simulink model "Modelo_bergman_mod_U"  (R2024b)
settings: Solver=VariableStepAuto  StartTime=0.0  StopTime=50000  RelTol=1e-3
undefined symbols (not defined in the file): n, p1, p2, p3, Vi
libraries: slpidlib x5
settings Model: Creator=USUARIO  LastModifiedBy=HP
settings SolverCC: AlgebraicLoopSolver=TrustRegion
settings DataIOCC: ReturnWorkspaceOutputs=off
settings DebuggingCC: UnconnectedInputMsg=warning  UnconnectedOutputMsg=warning  UnconnectedLineMsg=warning
settings ModelReferenceCC: EnableRefExpFcnMdlSchedulingChecks=on
settings RTWCC: GPUComputeCapability=3.5

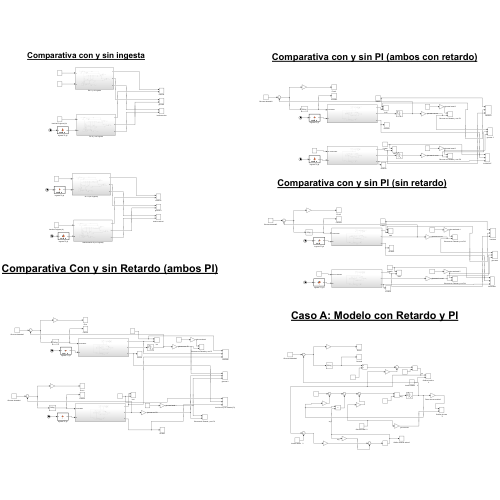
[thumbnail: Simulink's stored preview of the top-level diagram]
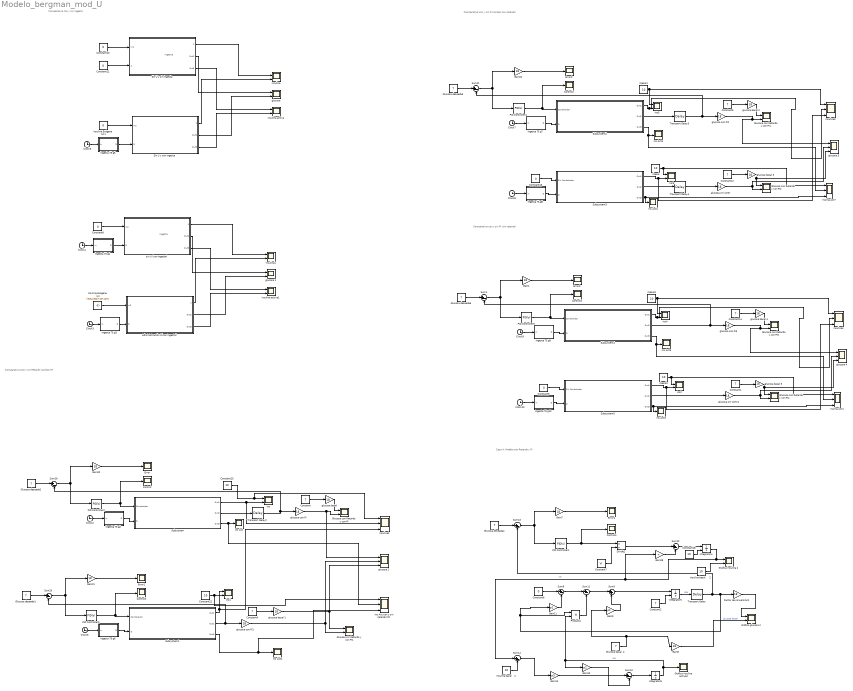
== system Modelo_bergman_mod_U ==
  note: Comparativa con y sin PI (ambos con retardo)
  note: Comparativa con y sin ingesta
  note: ingesta
  note: Comparativa Con y sin Retardo (ambos PI)
  note: Caso A: Modelo con Retardo y PI
  note: ingesta
  note: Comparativa con y sin PI (sin retardo)
  Administración U(con ingesta) : Subsystem
  Clock{2..10} (9 alike) : Clock
  Constant{,1..2,4..5,12,14} (7 alike) : Constant  Value=7
  Constant{3,6,8,10..11,13} (6 alike) : Constant  Value=0
  Constant18 : Constant  Value=10
  Constant22 : Constant  Value=10
  Constant23 : Constant  Value=10
  Constant7 : Constant  Value=Vi
  Control{,1..4} (5 alike) : Scope
  Divide2 : Product  Inputs=*/
  Error{,1..4} (5 alike) : Scope
  Factor de conversión2 : Gain  Gain=18
  Gain{1,7..8,20..22} (6 alike) : Gain  Gain=18
  Gain10 : Gain  Gain=p2
  Gain11 : Gain  Gain=p1
  Gain12 : Gain  Gain=p3
  Gain28 : Gain  Gain=n
  Gain9 : Gain  Gain=p1
  Glucosa basal  2 : Constant  Value=7
  Glucosa con Retardo y con PI{,1..4} (5 alike) : Scope  NumInputPorts=2
  Glucosa deseada{1..5} (5 alike) : Constant  Value=7
  Glucosa sin Retardo y con PI1 : Scope  NumInputPorts=2
  Gráfica glucosa 2 : Scope  NumInputPorts=2
  Gráfica insulina 2 : Scope  NumInputPorts=2
  Gráfica insulina activa2 : Scope
  Ingesta 75 g10 : MATLAB Function  TreatAsAtomicUnit=on
  Ingesta 75 g2 : MATLAB Function  TreatAsAtomicUnit=on
  Ingesta 75 g3 : MATLAB Function  TreatAsAtomicUnit=on
  Ingesta 75 g4 : MATLAB Function  TreatAsAtomicUnit=on
  Ingesta 75 g5 : MATLAB Function  TreatAsAtomicUnit=on
  Ingesta 75 g6 : MATLAB Function  TreatAsAtomicUnit=on
  Ingesta 75 g7 : MATLAB Function  TreatAsAtomicUnit=on
  Ingesta 75 g8 : MATLAB Function  TreatAsAtomicUnit=on
  Ingesta 75 g9 : MATLAB Function  TreatAsAtomicUnit=on
  Ins{,1..5} (6 alike) : Scope  NumInputPorts=2
  Ins Act{,1..5} (6 alike) : Scope
  Ins Act con y sin retardo (PI) : Scope  NumInputPorts=3
  Insulina Exógena (U) : Constant  Value=((5/54)/60)*10*12*5
  Insulina Exógena (U)1 : Constant  Value=0
  Insulina basal      2 : Constant  Value=10
  Insulina basal    2 : Constant  Value=10
  Integrator4 : Integrator  InitialConditionSource=external
  Integrator5 : Integrator  InitialConditionSource=external  InitialCondition=7
  Integrator6 : Integrator
  Inulina Act1 : Scope  NumInputPorts=3
  Inulina Act7 : Scope  NumInputPorts=3
  PID Controller1 : slpidlib/PID Controller  Controller=PID  Form=Parallel  TimeDomain=Continuous-time  UseExternalTs=off  SampleTime=-1  IntegratorMethod=Forward Euler  FilterMethod=Forward Euler  ControllerParametersSource=internal  P=-0.3195  I=-0.3195/2998.95  UseKiTs=off  D=0  UseExternalDerivativeSource=off  N=10  UseFilter=on  TunerSelectOption=Transfer Function Based (PID Tuner App)  InitialConditionSource=internal  InitialConditionForIntegrator=0  InitialConditionForFilter=0  DifferentiatorICPrevScaledInput=0  ExternalReset=none  TrackingMode=off  Kt=1  LimitOutput=off  SatLimitsSource=internal  UpperSaturationLimit=inf  LowerSaturationLimit=-inf  LinearizeAsGain=on  AntiWindupMode=none  Kb=1  LimitIntegrator=off  UpperIntegratorSaturationLimit=inf  LowerIntegratorSaturationLimit=-inf  POutMin=[]  POutMax=[]  IOutMin=[]  IOutMax=[]  DOutMin=[]  DOutMax=[]  NOutMin=[]  NOutMax=[]  SumOutMin=[]  SumOutMax=[]  SaturationOutMin=[]  SaturationOutMax=[]  PParamMin=[]  PParamMax=[]  IParamMin=[]  IParamMax=[]  DParamMin=[]  DParamMax=[]  NParamMin=[]  NParamMax=[]  KbParamMin=[]  KbParamMax=[]  KtParamMin=[]  KtParamMax=[]  KbOutMin=[]  KbOutMax=[]  KtOutMin=[]  KtOutMax=[]  IntegratorOutMin=[]  IntegratorOutMax=[]  FilterOutMin=[]  FilterOutMax=[]  SumI1OutMin=[]  SumI1OutMax=[]  SumI2OutMin=[]  SumI2OutMax=[]  SumI3OutMin=[]  SumI3OutMax=[]  SumI4OutMin=[]  SumI4OutMax=[]  SumDOutMin=[]  SumDOutMax=[]  DifferentiatorOutMin=[]  DifferentiatorOutMax=[]  FilterDiffOutCoefMin=[]  FilterDiffOutCoefMax=[]  ReciprocalOutMin=[]  ReciprocalOutMax=[]  SumDenOutMin=[]  SumDenOutMax=[]  SumNumOutMin=[]  SumNumOutMax=[]  DivideOutMin=[]  DivideOutMax=[]  UdiffTsProdOutMin=[]  UdiffTsProdOutMax=[]  NTsProdOutMin=[]  NTsProdOutMax=[]  UintegralTsProdOutMin=[]  UintegralTsProdOutMax=[]  UngainTsProdOutMin=[]  UngainTsProdOutMax=[]  ClampingZeroOutDataTypeStr=Inherit: Inherit via back propagation  ClampingZeroOutMin=[]  ClampingZeroOutMax=[]  FilterDenConstantOutDataTypeStr=Inherit: Inherit via back propagation  FilterDenConstantOutMin=[]  FilterDenConstantOutMax=[]  PCopyOutDataTypeStr=Inherit: Inherit via back propagation  PCopyOutMin=[]  PCopyOutMax=[]  NCopyOutDataTypeStr=Inherit: Inherit via back propagation  NCopyOutMin=[]  NCopyOutMax=[]  IntegratorContinuousStateAttributes=''  IntegratorStateMustResolveToSignalObject=off  IntegratorRTWStateStorageClass=Auto  FilterContinuousStateAttributes=''  FilterStateMustResolveToSignalObject=off  FilterRTWStateStorageClass=Auto  ParallelPVariant=InternalParameters  IdealPVariant=Disabled  IVariant=InternalParameters  DVariant=InternalParameters  IntegratorVariant=Continuous  SatVariant=Disabled  AWVariant=Passthrough  PCopyVariant=Disabled  TRVariant=Disabled  FdbkBlocksVariant=Forward  IdealPFdbkVariant=Disabled  SatFdbkVariant=Disabled  DerivativeFilterVariant=ContFilter  NVariant=InternalParameters  NCopyVariant=Disabled  FilterICVariant=InternalICsFilter  IntegratorICVariant=InternalICs  ExternalResetVariant=Disabled  TRSumVariant=Passthrough  SumFdbkVariant=Disabled  SumVariant=Sum_PID  TsampFilterVariant=InternalTs  TsampNgainVariant=Passthrough  TsampIntegralVariant=Disabled_SignalSpec  ExternalSaturationOutDataTypeStr=Inherit: Same as second input  DerivativeSourceVariant=ErrorSignal  PreIntVariant=InternalPreInt
  PID Controller2 : slpidlib/PID Controller  Controller=PID  Form=Parallel  TimeDomain=Continuous-time  UseExternalTs=off  SampleTime=-1  IntegratorMethod=Forward Euler  FilterMethod=Forward Euler  ControllerParametersSource=internal  P=-0.3195*0.3  I=-0.3195/2998.95*0.3  UseKiTs=off  D=0  UseExternalDerivativeSource=off  N=10  UseFilter=on  TunerSelectOption=Transfer Function Based (PID Tuner App)  InitialConditionSource=internal  InitialConditionForIntegrator=0  InitialConditionForFilter=0  DifferentiatorICPrevScaledInput=0  ExternalReset=none  TrackingMode=off  Kt=1  LimitOutput=off  SatLimitsSource=internal  UpperSaturationLimit=inf  LowerSaturationLimit=-inf  LinearizeAsGain=on  AntiWindupMode=none  Kb=1  LimitIntegrator=off  UpperIntegratorSaturationLimit=inf  LowerIntegratorSaturationLimit=-inf  POutMin=[]  POutMax=[]  IOutMin=[]  IOutMax=[]  DOutMin=[]  DOutMax=[]  NOutMin=[]  NOutMax=[]  SumOutMin=[]  SumOutMax=[]  SaturationOutMin=[]  SaturationOutMax=[]  PParamMin=[]  PParamMax=[]  IParamMin=[]  IParamMax=[]  DParamMin=[]  DParamMax=[]  NParamMin=[]  NParamMax=[]  KbParamMin=[]  KbParamMax=[]  KtParamMin=[]  KtParamMax=[]  KbOutMin=[]  KbOutMax=[]  KtOutMin=[]  KtOutMax=[]  IntegratorOutMin=[]  IntegratorOutMax=[]  FilterOutMin=[]  FilterOutMax=[]  SumI1OutMin=[]  SumI1OutMax=[]  SumI2OutMin=[]  SumI2OutMax=[]  SumI3OutMin=[]  SumI3OutMax=[]  SumI4OutMin=[]  SumI4OutMax=[]  SumDOutMin=[]  SumDOutMax=[]  DifferentiatorOutMin=[]  DifferentiatorOutMax=[]  FilterDiffOutCoefMin=[]  FilterDiffOutCoefMax=[]  ReciprocalOutMin=[]  ReciprocalOutMax=[]  SumDenOutMin=[]  SumDenOutMax=[]  SumNumOutMin=[]  SumNumOutMax=[]  DivideOutMin=[]  DivideOutMax=[]  UdiffTsProdOutMin=[]  UdiffTsProdOutMax=[]  NTsProdOutMin=[]  NTsProdOutMax=[]  UintegralTsProdOutMin=[]  UintegralTsProdOutMax=[]  UngainTsProdOutMin=[]  UngainTsProdOutMax=[]  ClampingZeroOutDataTypeStr=Inherit: Inherit via back propagation  ClampingZeroOutMin=[]  ClampingZeroOutMax=[]  FilterDenConstantOutDataTypeStr=Inherit: Inherit via back propagation  FilterDenConstantOutMin=[]  FilterDenConstantOutMax=[]  PCopyOutDataTypeStr=Inherit: Inherit via back propagation  PCopyOutMin=[]  PCopyOutMax=[]  NCopyOutDataTypeStr=Inherit: Inherit via back propagation  NCopyOutMin=[]  NCopyOutMax=[]  IntegratorContinuousStateAttributes=''  IntegratorStateMustResolveToSignalObject=off  IntegratorRTWStateStorageClass=Auto  FilterContinuousStateAttributes=''  FilterStateMustResolveToSignalObject=off  FilterRTWStateStorageClass=Auto  ParallelPVariant=InternalParameters  IdealPVariant=Disabled  IVariant=InternalParameters  DVariant=InternalParameters  IntegratorVariant=Continuous  SatVariant=Disabled  AWVariant=Passthrough  PCopyVariant=Disabled  TRVariant=Disabled  FdbkBlocksVariant=Forward  IdealPFdbkVariant=Disabled  SatFdbkVariant=Disabled  DerivativeFilterVariant=ContFilter  NVariant=InternalParameters  NCopyVariant=Disabled  FilterICVariant=InternalICsFilter  IntegratorICVariant=InternalICs  ExternalResetVariant=Disabled  TRSumVariant=Passthrough  SumFdbkVariant=Disabled  SumVariant=Sum_PID  TsampFilterVariant=InternalTs  TsampNgainVariant=Passthrough  TsampIntegralVariant=Disabled_SignalSpec  ExternalSaturationOutDataTypeStr=Inherit: Same as second input  DerivativeSourceVariant=ErrorSignal  PreIntVariant=InternalPreInt
  PID Controller3 : slpidlib/PID Controller  Controller=PID  Form=Parallel  TimeDomain=Continuous-time  UseExternalTs=off  SampleTime=-1  IntegratorMethod=Forward Euler  FilterMethod=Forward Euler  ControllerParametersSource=internal  P=-0.3195*0.3  I=-0.3195/2998.95*0.3  UseKiTs=off  D=0  UseExternalDerivativeSource=off  N=10  UseFilter=on  TunerSelectOption=Transfer Function Based (PID Tuner App)  InitialConditionSource=internal  InitialConditionForIntegrator=0  InitialConditionForFilter=0  DifferentiatorICPrevScaledInput=0  ExternalReset=none  TrackingMode=off  Kt=1  LimitOutput=off  SatLimitsSource=internal  UpperSaturationLimit=inf  LowerSaturationLimit=-inf  LinearizeAsGain=on  AntiWindupMode=none  Kb=1  LimitIntegrator=off  UpperIntegratorSaturationLimit=inf  LowerIntegratorSaturationLimit=-inf  POutMin=[]  POutMax=[]  IOutMin=[]  IOutMax=[]  DOutMin=[]  DOutMax=[]  NOutMin=[]  NOutMax=[]  SumOutMin=[]  SumOutMax=[]  SaturationOutMin=[]  SaturationOutMax=[]  PParamMin=[]  PParamMax=[]  IParamMin=[]  IParamMax=[]  DParamMin=[]  DParamMax=[]  NParamMin=[]  NParamMax=[]  KbParamMin=[]  KbParamMax=[]  KtParamMin=[]  KtParamMax=[]  KbOutMin=[]  KbOutMax=[]  KtOutMin=[]  KtOutMax=[]  IntegratorOutMin=[]  IntegratorOutMax=[]  FilterOutMin=[]  FilterOutMax=[]  SumI1OutMin=[]  SumI1OutMax=[]  SumI2OutMin=[]  SumI2OutMax=[]  SumI3OutMin=[]  SumI3OutMax=[]  SumI4OutMin=[]  SumI4OutMax=[]  SumDOutMin=[]  SumDOutMax=[]  DifferentiatorOutMin=[]  DifferentiatorOutMax=[]  FilterDiffOutCoefMin=[]  FilterDiffOutCoefMax=[]  ReciprocalOutMin=[]  ReciprocalOutMax=[]  SumDenOutMin=[]  SumDenOutMax=[]  SumNumOutMin=[]  SumNumOutMax=[]  DivideOutMin=[]  DivideOutMax=[]  UdiffTsProdOutMin=[]  UdiffTsProdOutMax=[]  NTsProdOutMin=[]  NTsProdOutMax=[]  UintegralTsProdOutMin=[]  UintegralTsProdOutMax=[]  UngainTsProdOutMin=[]  UngainTsProdOutMax=[]  ClampingZeroOutDataTypeStr=Inherit: Inherit via back propagation  ClampingZeroOutMin=[]  ClampingZeroOutMax=[]  FilterDenConstantOutDataTypeStr=Inherit: Inherit via back propagation  FilterDenConstantOutMin=[]  FilterDenConstantOutMax=[]  PCopyOutDataTypeStr=Inherit: Inherit via back propagation  PCopyOutMin=[]  PCopyOutMax=[]  NCopyOutDataTypeStr=Inherit: Inherit via back propagation  NCopyOutMin=[]  NCopyOutMax=[]  IntegratorContinuousStateAttributes=''  IntegratorStateMustResolveToSignalObject=off  IntegratorRTWStateStorageClass=Auto  FilterContinuousStateAttributes=''  FilterStateMustResolveToSignalObject=off  FilterRTWStateStorageClass=Auto  ParallelPVariant=InternalParameters  IdealPVariant=Disabled  IVariant=InternalParameters  DVariant=InternalParameters  IntegratorVariant=Continuous  SatVariant=Disabled  AWVariant=Passthrough  PCopyVariant=Disabled  TRVariant=Disabled  FdbkBlocksVariant=Forward  IdealPFdbkVariant=Disabled  SatFdbkVariant=Disabled  DerivativeFilterVariant=ContFilter  NVariant=InternalParameters  NCopyVariant=Disabled  FilterICVariant=InternalICsFilter  IntegratorICVariant=InternalICs  ExternalResetVariant=Disabled  TRSumVariant=Passthrough  SumFdbkVariant=Disabled  SumVariant=Sum_PID  TsampFilterVariant=InternalTs  TsampNgainVariant=Passthrough  TsampIntegralVariant=Disabled_SignalSpec  ExternalSaturationOutDataTypeStr=Inherit: Same as second input  DerivativeSourceVariant=ErrorSignal  PreIntVariant=InternalPreInt
  PID Controller4 : slpidlib/PID Controller  Controller=PID  Form=Parallel  TimeDomain=Continuous-time  UseExternalTs=off  SampleTime=-1  IntegratorMethod=Forward Euler  FilterMethod=Forward Euler  ControllerParametersSource=internal  P=-0.3195  I=-0.3195/2998.95  UseKiTs=off  D=0  UseExternalDerivativeSource=off  N=10  UseFilter=on  TunerSelectOption=Transfer Function Based (PID Tuner App)  InitialConditionSource=internal  InitialConditionForIntegrator=0  InitialConditionForFilter=0  DifferentiatorICPrevScaledInput=0  ExternalReset=none  TrackingMode=off  Kt=1  LimitOutput=off  SatLimitsSource=internal  UpperSaturationLimit=inf  LowerSaturationLimit=-inf  LinearizeAsGain=on  AntiWindupMode=none  Kb=1  LimitIntegrator=off  UpperIntegratorSaturationLimit=inf  LowerIntegratorSaturationLimit=-inf  POutMin=[]  POutMax=[]  IOutMin=[]  IOutMax=[]  DOutMin=[]  DOutMax=[]  NOutMin=[]  NOutMax=[]  SumOutMin=[]  SumOutMax=[]  SaturationOutMin=[]  SaturationOutMax=[]  PParamMin=[]  PParamMax=[]  IParamMin=[]  IParamMax=[]  DParamMin=[]  DParamMax=[]  NParamMin=[]  NParamMax=[]  KbParamMin=[]  KbParamMax=[]  KtParamMin=[]  KtParamMax=[]  KbOutMin=[]  KbOutMax=[]  KtOutMin=[]  KtOutMax=[]  IntegratorOutMin=[]  IntegratorOutMax=[]  FilterOutMin=[]  FilterOutMax=[]  SumI1OutMin=[]  SumI1OutMax=[]  SumI2OutMin=[]  SumI2OutMax=[]  SumI3OutMin=[]  SumI3OutMax=[]  SumI4OutMin=[]  SumI4OutMax=[]  SumDOutMin=[]  SumDOutMax=[]  DifferentiatorOutMin=[]  DifferentiatorOutMax=[]  FilterDiffOutCoefMin=[]  FilterDiffOutCoefMax=[]  ReciprocalOutMin=[]  ReciprocalOutMax=[]  SumDenOutMin=[]  SumDenOutMax=[]  SumNumOutMin=[]  SumNumOutMax=[]  DivideOutMin=[]  DivideOutMax=[]  UdiffTsProdOutMin=[]  UdiffTsProdOutMax=[]  NTsProdOutMin=[]  NTsProdOutMax=[]  UintegralTsProdOutMin=[]  UintegralTsProdOutMax=[]  UngainTsProdOutMin=[]  UngainTsProdOutMax=[]  ClampingZeroOutDataTypeStr=Inherit: Inherit via back propagation  ClampingZeroOutMin=[]  ClampingZeroOutMax=[]  FilterDenConstantOutDataTypeStr=Inherit: Inherit via back propagation  FilterDenConstantOutMin=[]  FilterDenConstantOutMax=[]  PCopyOutDataTypeStr=Inherit: Inherit via back propagation  PCopyOutMin=[]  PCopyOutMax=[]  NCopyOutDataTypeStr=Inherit: Inherit via back propagation  NCopyOutMin=[]  NCopyOutMax=[]  IntegratorContinuousStateAttributes=''  IntegratorStateMustResolveToSignalObject=off  IntegratorRTWStateStorageClass=Auto  FilterContinuousStateAttributes=''  FilterStateMustResolveToSignalObject=off  FilterRTWStateStorageClass=Auto  ParallelPVariant=InternalParameters  IdealPVariant=Disabled  IVariant=InternalParameters  DVariant=InternalParameters  IntegratorVariant=Continuous  SatVariant=Disabled  AWVariant=Passthrough  PCopyVariant=Disabled  TRVariant=Disabled  FdbkBlocksVariant=Forward  IdealPFdbkVariant=Disabled  SatFdbkVariant=Disabled  DerivativeFilterVariant=ContFilter  NVariant=InternalParameters  NCopyVariant=Disabled  FilterICVariant=InternalICsFilter  IntegratorICVariant=InternalICs  ExternalResetVariant=Disabled  TRSumVariant=Passthrough  SumFdbkVariant=Disabled  SumVariant=Sum_PID  TsampFilterVariant=InternalTs  TsampNgainVariant=Passthrough  TsampIntegralVariant=Disabled_SignalSpec  ExternalSaturationOutDataTypeStr=Inherit: Same as second input  DerivativeSourceVariant=ErrorSignal  PreIntVariant=InternalPreInt
  PID Controller5 : slpidlib/PID Controller  Controller=PID  Form=Parallel  TimeDomain=Continuous-time  UseExternalTs=off  SampleTime=-1  IntegratorMethod=Forward Euler  FilterMethod=Forward Euler  ControllerParametersSource=internal  P=-0.3195  I=-0.3195/2998.95  UseKiTs=off  D=0  UseExternalDerivativeSource=off  N=10  UseFilter=on  TunerSelectOption=Transfer Function Based (PID Tuner App)  InitialConditionSource=internal  InitialConditionForIntegrator=0  InitialConditionForFilter=0  DifferentiatorICPrevScaledInput=0  ExternalReset=none  TrackingMode=off  Kt=1  LimitOutput=off  SatLimitsSource=internal  UpperSaturationLimit=inf  LowerSaturationLimit=-inf  LinearizeAsGain=on  AntiWindupMode=none  Kb=1  LimitIntegrator=off  UpperIntegratorSaturationLimit=inf  LowerIntegratorSaturationLimit=-inf  POutMin=[]  POutMax=[]  IOutMin=[]  IOutMax=[]  DOutMin=[]  DOutMax=[]  NOutMin=[]  NOutMax=[]  SumOutMin=[]  SumOutMax=[]  SaturationOutMin=[]  SaturationOutMax=[]  PParamMin=[]  PParamMax=[]  IParamMin=[]  IParamMax=[]  DParamMin=[]  DParamMax=[]  NParamMin=[]  NParamMax=[]  KbParamMin=[]  KbParamMax=[]  KtParamMin=[]  KtParamMax=[]  KbOutMin=[]  KbOutMax=[]  KtOutMin=[]  KtOutMax=[]  IntegratorOutMin=[]  IntegratorOutMax=[]  FilterOutMin=[]  FilterOutMax=[]  SumI1OutMin=[]  SumI1OutMax=[]  SumI2OutMin=[]  SumI2OutMax=[]  SumI3OutMin=[]  SumI3OutMax=[]  SumI4OutMin=[]  SumI4OutMax=[]  SumDOutMin=[]  SumDOutMax=[]  DifferentiatorOutMin=[]  DifferentiatorOutMax=[]  FilterDiffOutCoefMin=[]  FilterDiffOutCoefMax=[]  ReciprocalOutMin=[]  ReciprocalOutMax=[]  SumDenOutMin=[]  SumDenOutMax=[]  SumNumOutMin=[]  SumNumOutMax=[]  DivideOutMin=[]  DivideOutMax=[]  UdiffTsProdOutMin=[]  UdiffTsProdOutMax=[]  NTsProdOutMin=[]  NTsProdOutMax=[]  UintegralTsProdOutMin=[]  UintegralTsProdOutMax=[]  UngainTsProdOutMin=[]  UngainTsProdOutMax=[]  ClampingZeroOutDataTypeStr=Inherit: Inherit via back propagation  ClampingZeroOutMin=[]  ClampingZeroOutMax=[]  FilterDenConstantOutDataTypeStr=Inherit: Inherit via back propagation  FilterDenConstantOutMin=[]  FilterDenConstantOutMax=[]  PCopyOutDataTypeStr=Inherit: Inherit via back propagation  PCopyOutMin=[]  PCopyOutMax=[]  NCopyOutDataTypeStr=Inherit: Inherit via back propagation  NCopyOutMin=[]  NCopyOutMax=[]  IntegratorContinuousStateAttributes=''  IntegratorStateMustResolveToSignalObject=off  IntegratorRTWStateStorageClass=Auto  FilterContinuousStateAttributes=''  FilterStateMustResolveToSignalObject=off  FilterRTWStateStorageClass=Auto  ParallelPVariant=InternalParameters  IdealPVariant=Disabled  IVariant=InternalParameters  DVariant=InternalParameters  IntegratorVariant=Continuous  SatVariant=Disabled  AWVariant=Passthrough  PCopyVariant=Disabled  TRVariant=Disabled  FdbkBlocksVariant=Forward  IdealPFdbkVariant=Disabled  SatFdbkVariant=Disabled  DerivativeFilterVariant=ContFilter  NVariant=InternalParameters  NCopyVariant=Disabled  FilterICVariant=InternalICsFilter  IntegratorICVariant=InternalICs  ExternalResetVariant=Disabled  TRSumVariant=Passthrough  SumFdbkVariant=Disabled  SumVariant=Sum_PID  TsampFilterVariant=InternalTs  TsampNgainVariant=Passthrough  TsampIntegralVariant=Disabled_SignalSpec  ExternalSaturationOutDataTypeStr=Inherit: Same as second input  DerivativeSourceVariant=ErrorSignal  PreIntVariant=InternalPreInt
  Product2 : Product
  Sin U y con Ingesta : Subsystem
  Sin U y sin ingesta : Subsystem
  Subsystem : Subsystem
  Subsystem1 : Subsystem
  Subsystem2 : Subsystem
  Subsystem3 : Subsystem
  Subsystem4 : Subsystem
  Subsystem5 : Subsystem
  Sum{1,8,10..14,20..21,29} (10 alike) : Sum  Inputs=|+-
  Sum9 : Sum  Inputs=|++
  Transport Delay : TransportDelay  DelayTime=900
  Transport Delay2 : TransportDelay  DelayTime=900  InitialOutput=7
  Transport Delay3 : TransportDelay  DelayTime=600  InitialOutput=7
  Transport Delay4 : TransportDelay  DelayTime=600  InitialOutput=7
  "glucosa " : Scope  NumInputPorts=2
  glucosa 1 : Scope  NumInputPorts=2
  glucosa 2 : Scope  NumInputPorts=3
  glucosa 3 : Scope  NumInputPorts=3
  glucosa 4 : Scope  NumInputPorts=3
  glucosa basal {,1..5} (6 alike) : Gain  Gain=18
  glucosa con PI{,1..3} (4 alike) : Gain  Gain=18
  glucosa sin contr : Gain  Gain=18
  glucosa sin contr1 : Gain  Gain=18
  i basal{,1..3} (4 alike) : Constant  Value=10
  insulina : Scope  NumInputPorts=2
  insulina activa : Scope  NumInputPorts=2
  insulina activa1 : Scope  NumInputPorts=2
  insulina1 : Scope  NumInputPorts=2
  insulina2 : Scope  NumInputPorts=3
  insulina3 : Scope  NumInputPorts=3
  insulina4 : Scope  NumInputPorts=3
  sin U (con Ingesta) : Subsystem
  wires:
  Constant6/1 -> Sum8/1
  Divide2/1 -> Sum12/1
  Gain11/1 -> Sum8/2
  Product2/1 -> Sum11/2
  Factor de conversión2/1 -> Gráfica glucosa 2/1
  Glucosa basal  2/1 -> Gain9/1, Gain8/1
  Sum10/1 -> Integrator6/1
  Constant18/1 -> Integrator4/2
  Glucosa deseada4/1 -> Sum13/1
  PID Controller1/1 -> Control4/1, Divide2/1
  Sum8/1 -> Sum11/1
  Gain8/1 -> Gráfica glucosa 2/2  "glucosa basal"
  Sum11/1 -> Sum9/1
  Sum13/1 -> PID Controller1/1, Gain7/1
  Insulina basal    2/1 -> Sum14/2
  Sum9/1 -> Integrator5/1
  Integrator4/1 -> Gráfica insulina 2/1, Sum14/1, Gain28/1  "I(t)"
  Integrator5/1 -> Transport Delay/1  "G(t)"
  Insulina basal      2/1 -> Gráfica insulina 2/2
  Gain10/1 -> Sum10/2
  Sum14/1 -> Gain12/1
  Sum12/1 -> Integrator4/1
  Gain7/1 -> Error4/1
  Gain12/1 -> Sum10/1
  Integrator6/1 -> Product2/2, Gain10/1, Gráfica insulina activa2/1  "X(t)"
  Constant7/1 -> Divide2/2
  Constant2/1 -> Integrator5/2
  Gain28/1 -> Sum12/2
  Gain9/1 -> Sum9/2
  Constant8/1 -> sin U (con Ingesta)/1(In2)
  Insulina Exógena (U)/1 -> Administración U(con ingesta)/1(In2)
  sin U (con Ingesta)/2(Out2) -> glucosa 1/1
  Administración U(con ingesta)/2(Out2) -> glucosa 1/2
  Administración U(con ingesta)/1(1) -> insulina1/2
  sin U (con Ingesta)/1(1) -> insulina1/1
  Clock4/1 -> Ingesta 75 g4/1(in)
  Ingesta 75 g3/1(D) -> Administración U(con ingesta)/2(D)
  Clock3/1 -> Ingesta 75 g3/1(in)
  Ingesta 75 g4/1(D) -> sin U (con Ingesta)/2(D)
  Administración U(con ingesta)/3(Out3) -> insulina activa1/2
  sin U (con Ingesta)/3(Out3) -> insulina activa1/1
  Sin U y sin ingesta/3(Out3) -> insulina activa/1
  Sin U y con Ingesta/1(1) -> insulina/2
  Ingesta 75 g5/1(D) -> Sin U y con Ingesta/2(D)
  Sin U y con Ingesta/3(Out3) -> insulina activa/2
  Constant10/1 -> Sin U y sin ingesta/1(In2)
  Insulina Exógena (U)1/1 -> Sin U y con Ingesta/1(In2)
  Clock5/1 -> Ingesta 75 g5/1(in)
  Sin U y sin ingesta/1(1) -> insulina/1
  Sin U y con Ingesta/2(Out2) -> "glucosa "/2
  Sin U y sin ingesta/2(Out2) -> "glucosa "/1
  Constant11/1 -> Sin U y sin ingesta/2(2)
  Clock2/1 -> Ingesta 75 g2/1(in)
  Ingesta 75 g2/1(D) -> Subsystem/2(D)
  PID Controller2/1 -> Control/1, Subsystem/1(Controlador)
  Glucosa deseada2/1 -> Sum29/1
  Gain20/1 -> Error/1
  Sum29/1 -> PID Controller2/1, Gain20/1
  Transport Delay2/1 -> Sum29/2, glucosa con PI/1
  glucosa con PI/1 -> glucosa 2/1, Glucosa con Retardo y con PI/2
  Subsystem/2(Out2) -> Transport Delay2/1
  Constant/1 -> "glucosa basal "/1
  "glucosa basal "/1 -> Glucosa con Retardo y con PI/1
  PID Controller3/1 -> Control1/1, Subsystem1/1(Controlador)
  Gain21/1 -> Error1/1
  Constant4/1 -> glucosa basal 1/1
  glucosa con PI1/1 -> glucosa 2/2, Glucosa sin Retardo y con PI1/2
  Sum20/1 -> PID Controller3/1, Gain21/1
  Glucosa deseada1/1 -> Sum20/1
  glucosa basal 1/1 -> glucosa 2/3, Glucosa sin Retardo y con PI1/1
  Clock6/1 -> Ingesta 75 g6/1(in)
  Ingesta 75 g6/1(D) -> Subsystem1/2(D)
  Subsystem1/2(Out2) -> Sum20/2, glucosa con PI1/1
  PID Controller4/1 -> Control2/1, Subsystem2/1(Controlador)
  Gain22/1 -> Error2/1
  Constant5/1 -> glucosa basal 2/1
  glucosa con PI2/1 -> glucosa 3/1, Glucosa con Retardo y con PI1/2
  Sum21/1 -> PID Controller4/1, Gain22/1
  Transport Delay3/1 -> Sum21/2, glucosa con PI2/1
  Subsystem2/2(Out2) -> Transport Delay3/1
  Glucosa deseada3/1 -> Sum21/1
  glucosa basal 2/1 -> Glucosa con Retardo y con PI1/1
  Clock7/1 -> Ingesta 75 g7/1(in)
  Ingesta 75 g7/1(D) -> Subsystem2/2(D)
  Constant12/1 -> glucosa basal 3/1
  glucosa sin contr/1 -> glucosa 3/2, Glucosa con Retardo y con PI2/2
  Transport Delay4/1 -> glucosa sin contr/1
  Subsystem3/2(Out2) -> Transport Delay4/1
  glucosa basal 3/1 -> glucosa 3/3, Glucosa con Retardo y con PI2/1
  Clock8/1 -> Ingesta 75 g8/1(in)
  Ingesta 75 g8/1(D) -> Subsystem3/2(D)
  Constant13/1 -> Subsystem3/1(Sin Controlador)
  Subsystem/3(Out3) -> Ins Act con y sin retardo (PI)/2, Ins Act/1
  Subsystem/1(Out1) -> insulina2/2, Ins/2
  Subsystem1/1(Out1) -> insulina2/3, Ins1/1
  Subsystem1/3(Out3) -> Ins Act1/1, Ins Act con y sin retardo (PI)/3
  Constant22/1 -> Ins Act con y sin retardo (PI)/1, Ins1/2
  Constant23/1 -> insulina2/1, Ins/1
  Subsystem2/1(Out1) -> insulina3/2, Ins5/2
  Subsystem2/3(Out3) -> Inulina Act7/2, Ins Act4/1
  Subsystem3/1(Out1) -> insulina3/3, Ins3/2
  Subsystem3/3(Out3) -> Inulina Act7/3, Ins Act2/1
  i basal/1 -> Ins3/1, Inulina Act7/1
  i basal1/1 -> insulina3/1, Ins5/1
  Subsystem4/1(Out1) -> insulina4/2, Ins4/2
  glucosa con PI3/1 -> glucosa 4/1, Glucosa con Retardo y con PI3/2
  glucosa basal 5/1 -> glucosa 4/3, Glucosa con Retardo y con PI4/1
  i basal3/1 -> insulina4/1, Ins4/1
  Subsystem5/2(Out2) -> glucosa sin contr1/1
  Glucosa deseada5/1 -> Sum1/1
  Subsystem4/3(Out3) -> Inulina Act1/2, Ins Act5/1
  Subsystem4/2(Out2) -> Sum1/2, glucosa con PI3/1
  Subsystem5/1(Out1) -> insulina4/3, Ins2/2
  Gain1/1 -> Error3/1
  Sum1/1 -> PID Controller5/1, Gain1/1
  Constant1/1 -> glucosa basal 5/1
  i basal2/1 -> Ins2/1, Inulina Act1/1
  glucosa sin contr1/1 -> glucosa 4/2, Glucosa con Retardo y con PI4/2
  Clock9/1 -> Ingesta 75 g9/1(in)
  PID Controller5/1 -> Control3/1, Subsystem4/1(Controlador)
  Ingesta 75 g9/1(D) -> Subsystem4/2(D)
  Clock10/1 -> Ingesta 75 g10/1(in)
  Subsystem5/3(Out3) -> Inulina Act1/3, Ins Act3/1
  Constant14/1 -> glucosa basal 4/1
  Constant3/1 -> Subsystem5/1(Sin Controlador)
  Ingesta 75 g10/1(D) -> Subsystem5/2(D)
  glucosa basal 4/1 -> Glucosa con Retardo y con PI3/1
  Transport Delay/1 -> Sum13/2, Factor de conversión2/1, Gain11/1, Product2/1

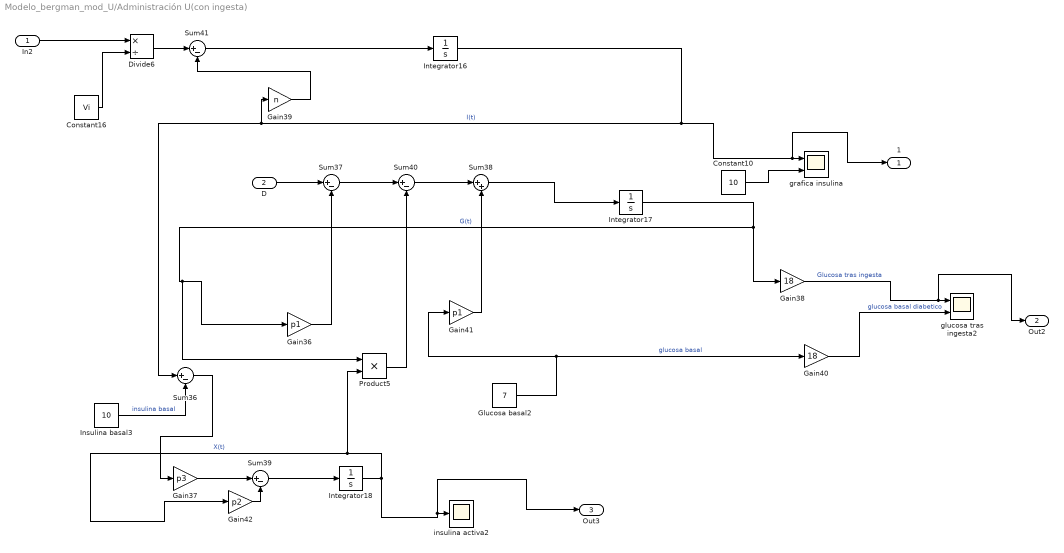
== system Modelo_bergman_mod_U/Administración U(con ingesta) ==
  In2 : Inport
  D : Inport  Port=2
  Constant10 : Constant  Value=10
  Constant16 : Constant  Value=Vi
  Divide6 : Product  Inputs=*/
  Gain36 : Gain  Gain=p1
  Gain37 : Gain  Gain=p3
  Gain38 : Gain  Gain=18
  Gain39 : Gain  Gain=n
  Gain40 : Gain  Gain=18
  Gain41 : Gain  Gain=p1
  Gain42 : Gain  Gain=p2
  Glucosa basal2 : Constant  Value=7
  Insulina basal3 : Constant  Value=10
  Integrator16 : Integrator  InitialCondition=10
  Integrator17 : Integrator  InitialCondition=7
  Integrator18 : Integrator
  Product5 : Product
  Sum{36..37,39..41} (5 alike) : Sum  Inputs=|+-
  Sum38 : Sum  Inputs=|++
  glucosa tras ingesta2 : Scope  NumInputPorts=2
  grafica insulina : Scope  NumInputPorts=2
  insulina activa2 : Scope
  1 : Outport
  Out2 : Outport  Port=2
  Out3 : Outport  Port=3
  wires:
  Integrator18/1 -> Out3/1, insulina activa2/1, Product5/2, Gain42/1  "X(t)"
  Integrator17/1 -> Gain38/1, Product5/1, Gain36/1  "G(t)"
  Gain39/1 -> Sum41/2
  Glucosa basal2/1 -> Gain41/1, Gain40/1  "glucosa basal"
  Integrator16/1 -> Sum36/1, Gain39/1, 1/1, grafica insulina/1  "I(t)"
  Constant10/1 -> grafica insulina/2
  Gain42/1 -> Sum39/2
  D/1 -> Sum37/1
  Sum37/1 -> Sum40/1
  Sum39/1 -> Integrator18/1
  Gain40/1 -> glucosa tras ingesta2/2  "glucosa basal diabetico"
  Sum40/1 -> Sum38/1
  In2/1 -> Divide6/1
  Gain36/1 -> Sum37/2
  Gain38/1 -> Out2/1, glucosa tras ingesta2/1  "Glucosa tras ingesta"
  Sum36/1 -> Gain37/1
  Gain41/1 -> Sum38/2
  Gain37/1 -> Sum39/1
  Sum41/1 -> Integrator16/1
  Sum38/1 -> Integrator17/1
  Insulina basal3/1 -> Sum36/2  "insulina basal"
  Divide6/1 -> Sum41/1
  Constant16/1 -> Divide6/2
  Product5/1 -> Sum40/2

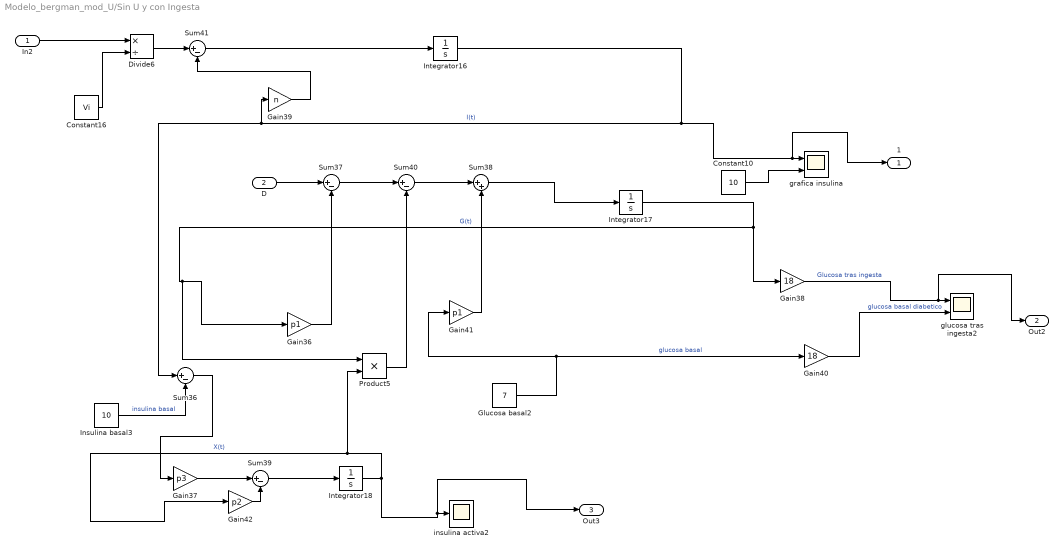
== system Modelo_bergman_mod_U/Sin U y con Ingesta ==
  In2 : Inport
  D : Inport  Port=2
  Constant10 : Constant  Value=10
  Constant16 : Constant  Value=Vi
  Divide6 : Product  Inputs=*/
  Gain36 : Gain  Gain=p1
  Gain37 : Gain  Gain=p3
  Gain38 : Gain  Gain=18
  Gain39 : Gain  Gain=n
  Gain40 : Gain  Gain=18
  Gain41 : Gain  Gain=p1
  Gain42 : Gain  Gain=p2
  Glucosa basal2 : Constant  Value=7
  Insulina basal3 : Constant  Value=10
  Integrator16 : Integrator  InitialCondition=10
  Integrator17 : Integrator  InitialCondition=7
  Integrator18 : Integrator
  Product5 : Product
  Sum{36..37,39..41} (5 alike) : Sum  Inputs=|+-
  Sum38 : Sum  Inputs=|++
  glucosa tras ingesta2 : Scope  NumInputPorts=2
  grafica insulina : Scope  NumInputPorts=2
  insulina activa2 : Scope
  1 : Outport
  Out2 : Outport  Port=2
  Out3 : Outport  Port=3
  wires:
  Integrator18/1 -> Out3/1, insulina activa2/1, Product5/2, Gain42/1  "X(t)"
  Integrator17/1 -> Gain38/1, Product5/1, Gain36/1  "G(t)"
  Gain39/1 -> Sum41/2
  Glucosa basal2/1 -> Gain41/1, Gain40/1  "glucosa basal"
  Integrator16/1 -> Sum36/1, Gain39/1, 1/1, grafica insulina/1  "I(t)"
  Constant10/1 -> grafica insulina/2
  Gain42/1 -> Sum39/2
  D/1 -> Sum37/1
  Sum37/1 -> Sum40/1
  Sum39/1 -> Integrator18/1
  Gain40/1 -> glucosa tras ingesta2/2  "glucosa basal diabetico"
  Sum40/1 -> Sum38/1
  In2/1 -> Divide6/1
  Gain36/1 -> Sum37/2
  Gain38/1 -> Out2/1, glucosa tras ingesta2/1  "Glucosa tras ingesta"
  Sum36/1 -> Gain37/1
  Gain41/1 -> Sum38/2
  Gain37/1 -> Sum39/1
  Sum41/1 -> Integrator16/1
  Sum38/1 -> Integrator17/1
  Insulina basal3/1 -> Sum36/2  "insulina basal"
  Divide6/1 -> Sum41/1
  Constant16/1 -> Divide6/2
  Product5/1 -> Sum40/2

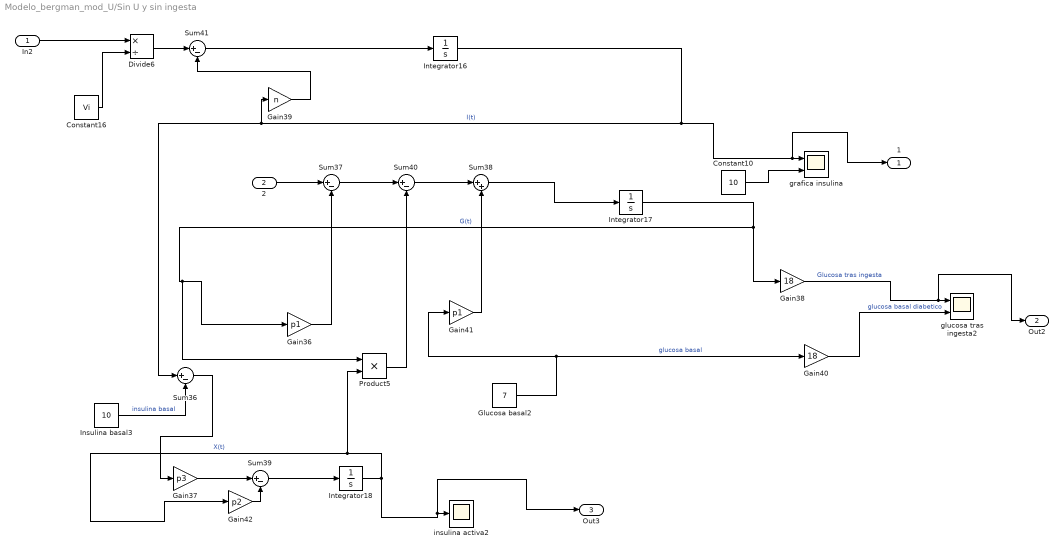
== system Modelo_bergman_mod_U/Sin U y sin ingesta ==
  In2 : Inport
  2 : Inport  Port=2
  Constant10 : Constant  Value=10
  Constant16 : Constant  Value=Vi
  Divide6 : Product  Inputs=*/
  Gain36 : Gain  Gain=p1
  Gain37 : Gain  Gain=p3
  Gain38 : Gain  Gain=18
  Gain39 : Gain  Gain=n
  Gain40 : Gain  Gain=18
  Gain41 : Gain  Gain=p1
  Gain42 : Gain  Gain=p2
  Glucosa basal2 : Constant  Value=7
  Insulina basal3 : Constant  Value=10
  Integrator16 : Integrator  InitialCondition=10
  Integrator17 : Integrator  InitialCondition=7
  Integrator18 : Integrator
  Product5 : Product
  Sum{36..37,39..41} (5 alike) : Sum  Inputs=|+-
  Sum38 : Sum  Inputs=|++
  glucosa tras ingesta2 : Scope  NumInputPorts=2
  grafica insulina : Scope  NumInputPorts=2
  insulina activa2 : Scope
  1 : Outport
  Out2 : Outport  Port=2
  Out3 : Outport  Port=3
  wires:
  Integrator18/1 -> Out3/1, insulina activa2/1, Product5/2, Gain42/1  "X(t)"
  Integrator17/1 -> Gain38/1, Product5/1, Gain36/1  "G(t)"
  Gain39/1 -> Sum41/2
  Glucosa basal2/1 -> Gain41/1, Gain40/1  "glucosa basal"
  Integrator16/1 -> Sum36/1, Gain39/1, 1/1, grafica insulina/1  "I(t)"
  Constant10/1 -> grafica insulina/2
  Gain42/1 -> Sum39/2
  2/1 -> Sum37/1
  Sum37/1 -> Sum40/1
  Sum39/1 -> Integrator18/1
  Gain40/1 -> glucosa tras ingesta2/2  "glucosa basal diabetico"
  Sum40/1 -> Sum38/1
  In2/1 -> Divide6/1
  Gain36/1 -> Sum37/2
  Gain38/1 -> Out2/1, glucosa tras ingesta2/1  "Glucosa tras ingesta"
  Sum36/1 -> Gain37/1
  Gain41/1 -> Sum38/2
  Gain37/1 -> Sum39/1
  Sum41/1 -> Integrator16/1
  Sum38/1 -> Integrator17/1
  Insulina basal3/1 -> Sum36/2  "insulina basal"
  Divide6/1 -> Sum41/1
  Constant16/1 -> Divide6/2
  Product5/1 -> Sum40/2

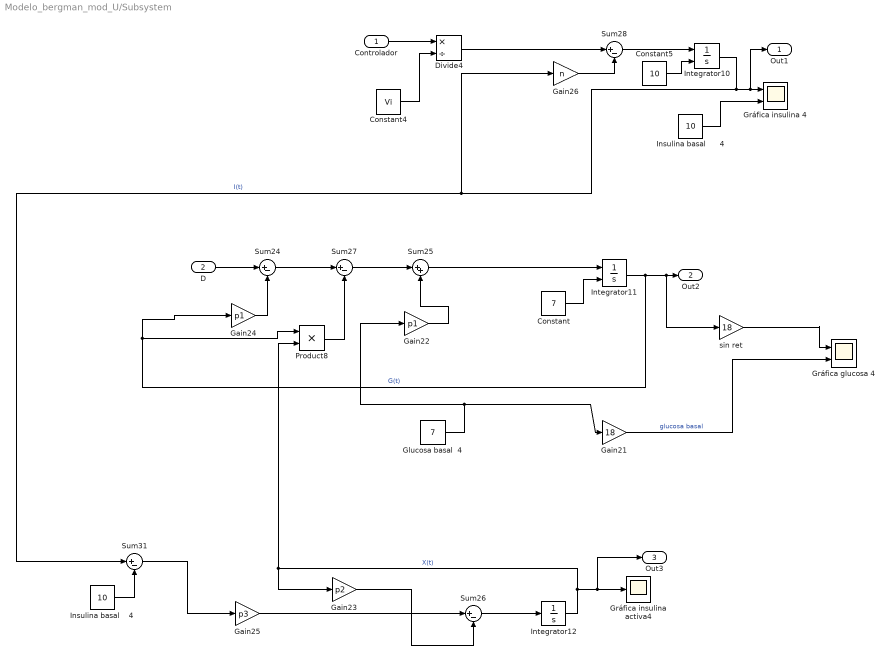
== system Modelo_bergman_mod_U/Subsystem ==
  Controlador : Inport
  D : Inport  Port=2
  Constant : Constant  Value=7
  Constant4 : Constant  Value=Vi
  Constant5 : Constant  Value=10
  Divide4 : Product  Inputs=*/
  Gain21 : Gain  Gain=18
  Gain22 : Gain  Gain=p1
  Gain23 : Gain  Gain=p2
  Gain24 : Gain  Gain=p1
  Gain25 : Gain  Gain=p3
  Gain26 : Gain  Gain=n
  Glucosa basal  4 : Constant  Value=7
  Gráfica glucosa 4 : Scope  NumInputPorts=2
  Gráfica insulina 4 : Scope  NumInputPorts=2
  Gráfica insulina activa4 : Scope
  Insulina basal      4 : Constant  Value=10
  Insulina basal    4 : Constant  Value=10
  Integrator10 : Integrator  InitialConditionSource=external
  Integrator11 : Integrator  InitialConditionSource=external  InitialCondition=7
  Integrator12 : Integrator
  Product8 : Product
  Sum{24,26..28,31} (5 alike) : Sum  Inputs=|+-
  Sum25 : Sum  Inputs=|++
  sin ret : Gain  Gain=18
  Out1 : Outport
  Out2 : Outport  Port=2
  Out3 : Outport  Port=3
  wires:
  Gain26/1 -> Sum28/2
  Glucosa basal  4/1 -> Gain22/1, Gain21/1
  D/1 -> Sum24/1
  Gain21/1 -> Gráfica glucosa 4/2  "glucosa basal"
  Integrator11/1 -> sin ret/1, Out2/1, Gain24/1, Product8/1  "G(t)"
  Integrator12/1 -> Product8/2, Gain23/1, Out3/1, Gráfica insulina activa4/1  "X(t)"
  Gain25/1 -> Sum26/1
  Integrator10/1 -> Out1/1, Gráfica insulina 4/1, Sum31/1, Gain26/1  "I(t)"
  Constant5/1 -> Integrator10/2
  Sum31/1 -> Gain25/1
  Sum26/1 -> Integrator12/1
  Gain23/1 -> Sum26/2
  Sum28/1 -> Integrator10/1
  Sum24/1 -> Sum27/1
  Sum25/1 -> Integrator11/1
  Gain24/1 -> Sum24/2
  Insulina basal      4/1 -> Gráfica insulina 4/2
  Sum27/1 -> Sum25/1
  Insulina basal    4/1 -> Sum31/2
  Divide4/1 -> Sum28/1
  Gain22/1 -> Sum25/2
  Product8/1 -> Sum27/2
  Constant4/1 -> Divide4/2
  Constant/1 -> Integrator11/2
  Controlador/1 -> Divide4/1
  sin ret/1 -> Gráfica glucosa 4/1

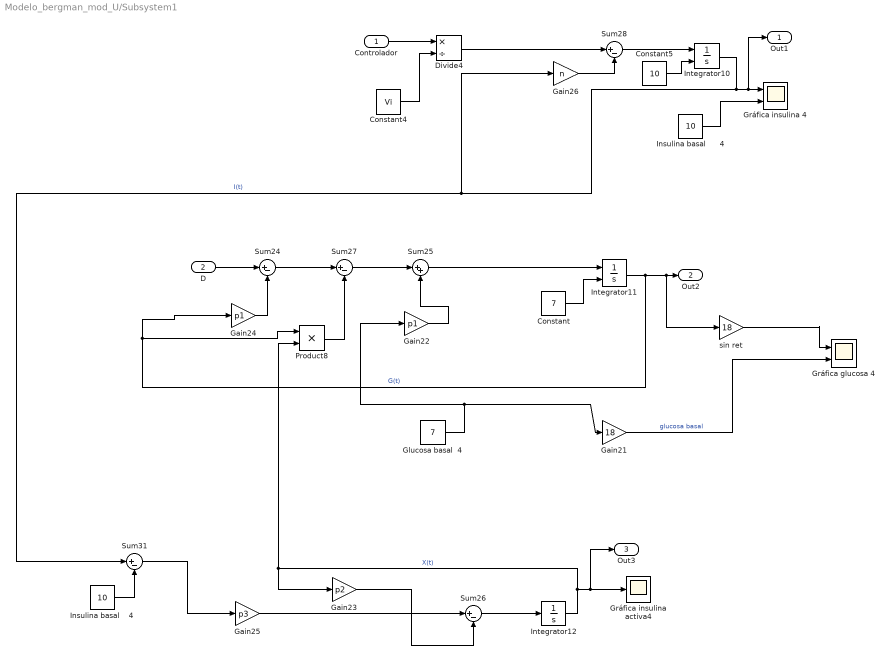
== system Modelo_bergman_mod_U/Subsystem1 ==
  Controlador : Inport
  D : Inport  Port=2
  Constant : Constant  Value=7
  Constant4 : Constant  Value=Vi
  Constant5 : Constant  Value=10
  Divide4 : Product  Inputs=*/
  Gain21 : Gain  Gain=18
  Gain22 : Gain  Gain=p1
  Gain23 : Gain  Gain=p2
  Gain24 : Gain  Gain=p1
  Gain25 : Gain  Gain=p3
  Gain26 : Gain  Gain=n
  Glucosa basal  4 : Constant  Value=7
  Gráfica glucosa 4 : Scope  NumInputPorts=2
  Gráfica insulina 4 : Scope  NumInputPorts=2
  Gráfica insulina activa4 : Scope
  Insulina basal      4 : Constant  Value=10
  Insulina basal    4 : Constant  Value=10
  Integrator10 : Integrator  InitialConditionSource=external
  Integrator11 : Integrator  InitialConditionSource=external  InitialCondition=7
  Integrator12 : Integrator
  Product8 : Product
  Sum{24,26..28,31} (5 alike) : Sum  Inputs=|+-
  Sum25 : Sum  Inputs=|++
  sin ret : Gain  Gain=18
  Out1 : Outport
  Out2 : Outport  Port=2
  Out3 : Outport  Port=3
  wires:
  Gain26/1 -> Sum28/2
  Glucosa basal  4/1 -> Gain22/1, Gain21/1
  D/1 -> Sum24/1
  Gain21/1 -> Gráfica glucosa 4/2  "glucosa basal"
  Integrator11/1 -> sin ret/1, Out2/1, Gain24/1, Product8/1  "G(t)"
  Integrator12/1 -> Product8/2, Gain23/1, Out3/1, Gráfica insulina activa4/1  "X(t)"
  Gain25/1 -> Sum26/1
  Integrator10/1 -> Out1/1, Gráfica insulina 4/1, Sum31/1, Gain26/1  "I(t)"
  Constant5/1 -> Integrator10/2
  Sum31/1 -> Gain25/1
  Sum26/1 -> Integrator12/1
  Gain23/1 -> Sum26/2
  Sum28/1 -> Integrator10/1
  Sum24/1 -> Sum27/1
  Sum25/1 -> Integrator11/1
  Gain24/1 -> Sum24/2
  Insulina basal      4/1 -> Gráfica insulina 4/2
  Sum27/1 -> Sum25/1
  Insulina basal    4/1 -> Sum31/2
  Divide4/1 -> Sum28/1
  Gain22/1 -> Sum25/2
  Product8/1 -> Sum27/2
  Constant4/1 -> Divide4/2
  Constant/1 -> Integrator11/2
  Controlador/1 -> Divide4/1
  sin ret/1 -> Gráfica glucosa 4/1

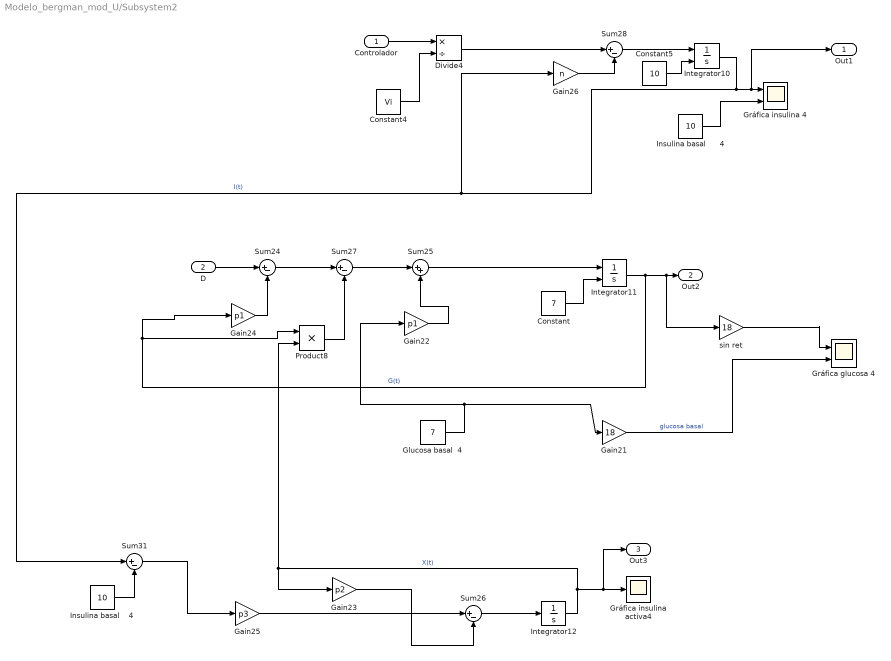
== system Modelo_bergman_mod_U/Subsystem2 ==
  Controlador : Inport
  D : Inport  Port=2
  Constant : Constant  Value=7
  Constant4 : Constant  Value=Vi
  Constant5 : Constant  Value=10
  Divide4 : Product  Inputs=*/
  Gain21 : Gain  Gain=18
  Gain22 : Gain  Gain=p1
  Gain23 : Gain  Gain=p2
  Gain24 : Gain  Gain=p1
  Gain25 : Gain  Gain=p3
  Gain26 : Gain  Gain=n
  Glucosa basal  4 : Constant  Value=7
  Gráfica glucosa 4 : Scope  NumInputPorts=2
  Gráfica insulina 4 : Scope  NumInputPorts=2
  Gráfica insulina activa4 : Scope
  Insulina basal      4 : Constant  Value=10
  Insulina basal    4 : Constant  Value=10
  Integrator10 : Integrator  InitialConditionSource=external
  Integrator11 : Integrator  InitialConditionSource=external  InitialCondition=7
  Integrator12 : Integrator
  Product8 : Product
  Sum{24,26..28,31} (5 alike) : Sum  Inputs=|+-
  Sum25 : Sum  Inputs=|++
  sin ret : Gain  Gain=18
  Out1 : Outport
  Out2 : Outport  Port=2
  Out3 : Outport  Port=3
  wires:
  Gain26/1 -> Sum28/2
  Glucosa basal  4/1 -> Gain22/1, Gain21/1
  D/1 -> Sum24/1
  Gain21/1 -> Gráfica glucosa 4/2  "glucosa basal"
  Integrator11/1 -> sin ret/1, Out2/1, Gain24/1, Product8/1  "G(t)"
  Integrator12/1 -> Product8/2, Gain23/1, Out3/1, Gráfica insulina activa4/1  "X(t)"
  Gain25/1 -> Sum26/1
  Integrator10/1 -> Out1/1, Gráfica insulina 4/1, Sum31/1, Gain26/1  "I(t)"
  Constant5/1 -> Integrator10/2
  Sum31/1 -> Gain25/1
  Sum26/1 -> Integrator12/1
  Gain23/1 -> Sum26/2
  Sum28/1 -> Integrator10/1
  Sum24/1 -> Sum27/1
  Sum25/1 -> Integrator11/1
  Gain24/1 -> Sum24/2
  Insulina basal      4/1 -> Gráfica insulina 4/2
  Sum27/1 -> Sum25/1
  Insulina basal    4/1 -> Sum31/2
  Divide4/1 -> Sum28/1
  Gain22/1 -> Sum25/2
  Product8/1 -> Sum27/2
  Constant4/1 -> Divide4/2
  Constant/1 -> Integrator11/2
  Controlador/1 -> Divide4/1
  sin ret/1 -> Gráfica glucosa 4/1

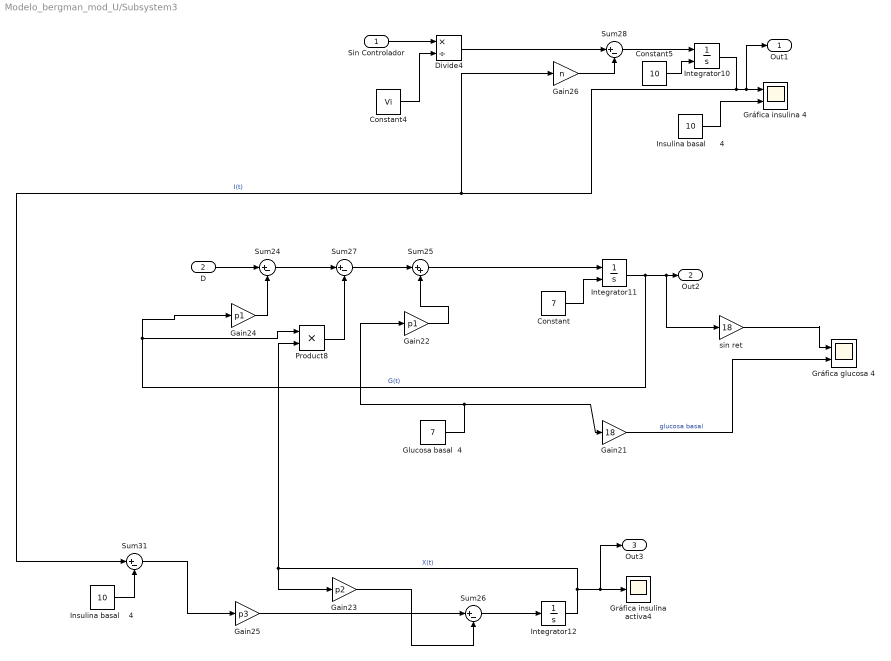
== system Modelo_bergman_mod_U/Subsystem3 ==
  Sin Controlador : Inport
  D : Inport  Port=2
  Constant : Constant  Value=7
  Constant4 : Constant  Value=Vi
  Constant5 : Constant  Value=10
  Divide4 : Product  Inputs=*/
  Gain21 : Gain  Gain=18
  Gain22 : Gain  Gain=p1
  Gain23 : Gain  Gain=p2
  Gain24 : Gain  Gain=p1
  Gain25 : Gain  Gain=p3
  Gain26 : Gain  Gain=n
  Glucosa basal  4 : Constant  Value=7
  Gráfica glucosa 4 : Scope  NumInputPorts=2
  Gráfica insulina 4 : Scope  NumInputPorts=2
  Gráfica insulina activa4 : Scope
  Insulina basal      4 : Constant  Value=10
  Insulina basal    4 : Constant  Value=10
  Integrator10 : Integrator  InitialConditionSource=external
  Integrator11 : Integrator  InitialConditionSource=external  InitialCondition=7
  Integrator12 : Integrator
  Product8 : Product
  Sum{24,26..28,31} (5 alike) : Sum  Inputs=|+-
  Sum25 : Sum  Inputs=|++
  sin ret : Gain  Gain=18
  Out1 : Outport
  Out2 : Outport  Port=2
  Out3 : Outport  Port=3
  wires:
  Gain26/1 -> Sum28/2
  Glucosa basal  4/1 -> Gain22/1, Gain21/1
  D/1 -> Sum24/1
  Gain21/1 -> Gráfica glucosa 4/2  "glucosa basal"
  Integrator11/1 -> sin ret/1, Out2/1, Gain24/1, Product8/1  "G(t)"
  Integrator12/1 -> Product8/2, Gain23/1, Out3/1, Gráfica insulina activa4/1  "X(t)"
  Gain25/1 -> Sum26/1
  Integrator10/1 -> Out1/1, Gráfica insulina 4/1, Sum31/1, Gain26/1  "I(t)"
  Constant5/1 -> Integrator10/2
  Sum31/1 -> Gain25/1
  Sum26/1 -> Integrator12/1
  Gain23/1 -> Sum26/2
  Sum28/1 -> Integrator10/1
  Sum24/1 -> Sum27/1
  Sum25/1 -> Integrator11/1
  Gain24/1 -> Sum24/2
  Insulina basal      4/1 -> Gráfica insulina 4/2
  Sum27/1 -> Sum25/1
  Insulina basal    4/1 -> Sum31/2
  Divide4/1 -> Sum28/1
  Gain22/1 -> Sum25/2
  Product8/1 -> Sum27/2
  Constant4/1 -> Divide4/2
  Constant/1 -> Integrator11/2
  Sin Controlador/1 -> Divide4/1
  sin ret/1 -> Gráfica glucosa 4/1

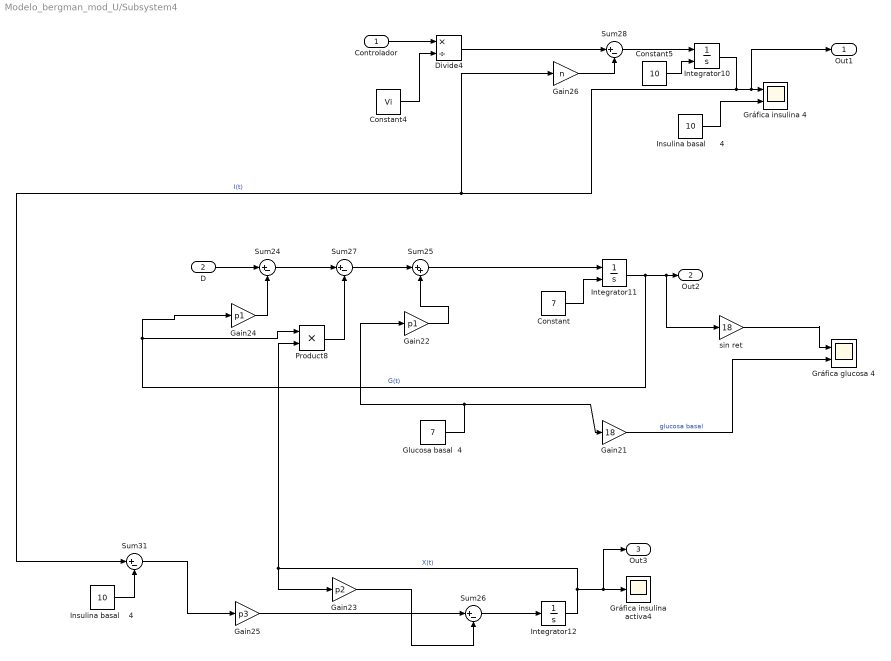
== system Modelo_bergman_mod_U/Subsystem4 ==
  Controlador : Inport
  D : Inport  Port=2
  Constant : Constant  Value=7
  Constant4 : Constant  Value=Vi
  Constant5 : Constant  Value=10
  Divide4 : Product  Inputs=*/
  Gain21 : Gain  Gain=18
  Gain22 : Gain  Gain=p1
  Gain23 : Gain  Gain=p2
  Gain24 : Gain  Gain=p1
  Gain25 : Gain  Gain=p3
  Gain26 : Gain  Gain=n
  Glucosa basal  4 : Constant  Value=7
  Gráfica glucosa 4 : Scope  NumInputPorts=2
  Gráfica insulina 4 : Scope  NumInputPorts=2
  Gráfica insulina activa4 : Scope
  Insulina basal      4 : Constant  Value=10
  Insulina basal    4 : Constant  Value=10
  Integrator10 : Integrator  InitialConditionSource=external
  Integrator11 : Integrator  InitialConditionSource=external  InitialCondition=7
  Integrator12 : Integrator
  Product8 : Product
  Sum{24,26..28,31} (5 alike) : Sum  Inputs=|+-
  Sum25 : Sum  Inputs=|++
  sin ret : Gain  Gain=18
  Out1 : Outport
  Out2 : Outport  Port=2
  Out3 : Outport  Port=3
  wires:
  Gain26/1 -> Sum28/2
  Glucosa basal  4/1 -> Gain22/1, Gain21/1
  D/1 -> Sum24/1
  Gain21/1 -> Gráfica glucosa 4/2  "glucosa basal"
  Integrator11/1 -> sin ret/1, Out2/1, Gain24/1, Product8/1  "G(t)"
  Integrator12/1 -> Product8/2, Gain23/1, Out3/1, Gráfica insulina activa4/1  "X(t)"
  Gain25/1 -> Sum26/1
  Integrator10/1 -> Out1/1, Gráfica insulina 4/1, Sum31/1, Gain26/1  "I(t)"
  Constant5/1 -> Integrator10/2
  Sum31/1 -> Gain25/1
  Sum26/1 -> Integrator12/1
  Gain23/1 -> Sum26/2
  Sum28/1 -> Integrator10/1
  Sum24/1 -> Sum27/1
  Sum25/1 -> Integrator11/1
  Gain24/1 -> Sum24/2
  Insulina basal      4/1 -> Gráfica insulina 4/2
  Sum27/1 -> Sum25/1
  Insulina basal    4/1 -> Sum31/2
  Divide4/1 -> Sum28/1
  Gain22/1 -> Sum25/2
  Product8/1 -> Sum27/2
  Constant4/1 -> Divide4/2
  Constant/1 -> Integrator11/2
  Controlador/1 -> Divide4/1
  sin ret/1 -> Gráfica glucosa 4/1

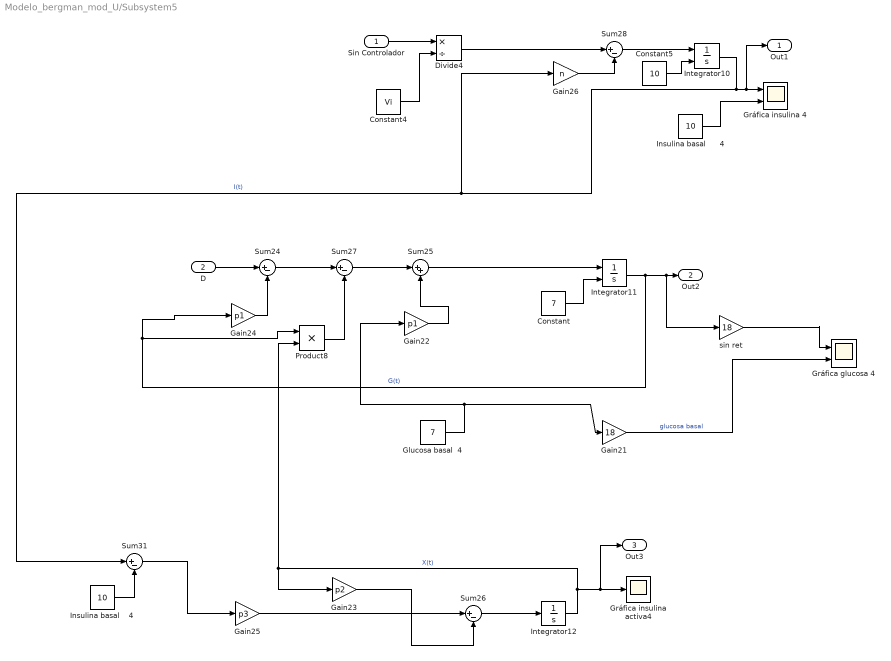
== system Modelo_bergman_mod_U/Subsystem5 ==
  Sin Controlador : Inport
  D : Inport  Port=2
  Constant : Constant  Value=7
  Constant4 : Constant  Value=Vi
  Constant5 : Constant  Value=10
  Divide4 : Product  Inputs=*/
  Gain21 : Gain  Gain=18
  Gain22 : Gain  Gain=p1
  Gain23 : Gain  Gain=p2
  Gain24 : Gain  Gain=p1
  Gain25 : Gain  Gain=p3
  Gain26 : Gain  Gain=n
  Glucosa basal  4 : Constant  Value=7
  Gráfica glucosa 4 : Scope  NumInputPorts=2
  Gráfica insulina 4 : Scope  NumInputPorts=2
  Gráfica insulina activa4 : Scope
  Insulina basal      4 : Constant  Value=10
  Insulina basal    4 : Constant  Value=10
  Integrator10 : Integrator  InitialConditionSource=external
  Integrator11 : Integrator  InitialConditionSource=external  InitialCondition=7
  Integrator12 : Integrator
  Product8 : Product
  Sum{24,26..28,31} (5 alike) : Sum  Inputs=|+-
  Sum25 : Sum  Inputs=|++
  sin ret : Gain  Gain=18
  Out1 : Outport
  Out2 : Outport  Port=2
  Out3 : Outport  Port=3
  wires:
  Gain26/1 -> Sum28/2
  Glucosa basal  4/1 -> Gain22/1, Gain21/1
  D/1 -> Sum24/1
  Gain21/1 -> Gráfica glucosa 4/2  "glucosa basal"
  Integrator11/1 -> sin ret/1, Out2/1, Gain24/1, Product8/1  "G(t)"
  Integrator12/1 -> Product8/2, Gain23/1, Out3/1, Gráfica insulina activa4/1  "X(t)"
  Gain25/1 -> Sum26/1
  Integrator10/1 -> Out1/1, Gráfica insulina 4/1, Sum31/1, Gain26/1  "I(t)"
  Constant5/1 -> Integrator10/2
  Sum31/1 -> Gain25/1
  Sum26/1 -> Integrator12/1
  Gain23/1 -> Sum26/2
  Sum28/1 -> Integrator10/1
  Sum24/1 -> Sum27/1
  Sum25/1 -> Integrator11/1
  Gain24/1 -> Sum24/2
  Insulina basal      4/1 -> Gráfica insulina 4/2
  Sum27/1 -> Sum25/1
  Insulina basal    4/1 -> Sum31/2
  Divide4/1 -> Sum28/1
  Gain22/1 -> Sum25/2
  Product8/1 -> Sum27/2
  Constant4/1 -> Divide4/2
  Constant/1 -> Integrator11/2
  Sin Controlador/1 -> Divide4/1
  sin ret/1 -> Gráfica glucosa 4/1

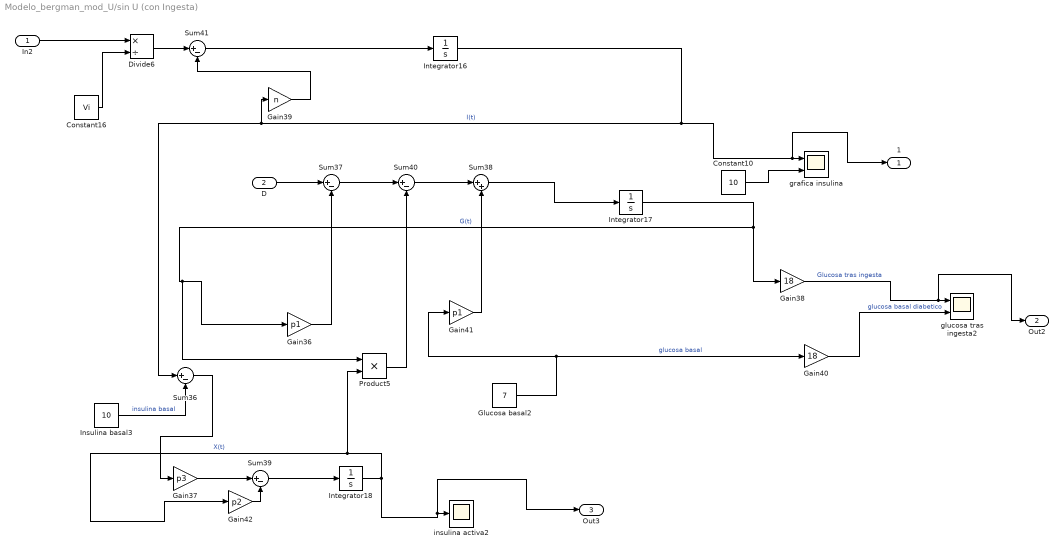
== system Modelo_bergman_mod_U/sin U (con Ingesta) ==
  In2 : Inport
  D : Inport  Port=2
  Constant10 : Constant  Value=10
  Constant16 : Constant  Value=Vi
  Divide6 : Product  Inputs=*/
  Gain36 : Gain  Gain=p1
  Gain37 : Gain  Gain=p3
  Gain38 : Gain  Gain=18
  Gain39 : Gain  Gain=n
  Gain40 : Gain  Gain=18
  Gain41 : Gain  Gain=p1
  Gain42 : Gain  Gain=p2
  Glucosa basal2 : Constant  Value=7
  Insulina basal3 : Constant  Value=10
  Integrator16 : Integrator  InitialCondition=10
  Integrator17 : Integrator  InitialCondition=7
  Integrator18 : Integrator
  Product5 : Product
  Sum{36..37,39..41} (5 alike) : Sum  Inputs=|+-
  Sum38 : Sum  Inputs=|++
  glucosa tras ingesta2 : Scope  NumInputPorts=2
  grafica insulina : Scope  NumInputPorts=2
  insulina activa2 : Scope
  1 : Outport
  Out2 : Outport  Port=2
  Out3 : Outport  Port=3
  wires:
  Integrator18/1 -> Out3/1, insulina activa2/1, Product5/2, Gain42/1  "X(t)"
  Integrator17/1 -> Gain38/1, Product5/1, Gain36/1  "G(t)"
  Gain39/1 -> Sum41/2
  Glucosa basal2/1 -> Gain41/1, Gain40/1  "glucosa basal"
  Integrator16/1 -> Sum36/1, Gain39/1, 1/1, grafica insulina/1  "I(t)"
  Constant10/1 -> grafica insulina/2
  Gain42/1 -> Sum39/2
  D/1 -> Sum37/1
  Sum37/1 -> Sum40/1
  Sum39/1 -> Integrator18/1
  Gain40/1 -> glucosa tras ingesta2/2  "glucosa basal diabetico"
  Sum40/1 -> Sum38/1
  In2/1 -> Divide6/1
  Gain36/1 -> Sum37/2
  Gain38/1 -> Out2/1, glucosa tras ingesta2/1  "Glucosa tras ingesta"
  Sum36/1 -> Gain37/1
  Gain41/1 -> Sum38/2
  Gain37/1 -> Sum39/1
  Sum41/1 -> Integrator16/1
  Sum38/1 -> Integrator17/1
  Insulina basal3/1 -> Sum36/2  "insulina basal"
  Divide6/1 -> Sum41/1
  Constant16/1 -> Divide6/2
  Product5/1 -> Sum40/2

== matlab function Modelo_bergman_mod_U/Ingesta 75 g3 ==
  data: in input; D output
function D = comida(in)
% Variables de entrada en la funcion
t = in(1) %- 8*60*60; % Ajuste para iniciar a las 8 de la mañana
 
% Parámetros del modelo
Ag = 0.8; % adimensional
Tmaxi = 55*60; % s
Vg = 13.79; % L
Tmaxg = 40*60; % s
t1 = 0;
Dg = 0;
f = 1000/180; % factor de conversión de g a mmol
 
% Comidas (perturbaciones) a lo largo de un día
Dg = 50*f;
% Ecuación
D = (Dg*Ag*(t-t1)*exp(-(t-t1)/Tmaxi))/(Vg*Tmaxg^2);

== matlab function Modelo_bergman_mod_U/Ingesta 75 g4 ==
  data: in input; D output
function D = comida(in)
% Variables de entrada en la funcion
t = in(1) %- 8*60*60; % Ajuste para iniciar a las 8 de la mañana
 
% Parámetros del modelo
Ag = 0.8; % adimensional
Tmaxi = 55*60; % s
Vg = 13.79; % L
Tmaxg = 40*60; % s
t1 = 0;
Dg = 0;
f = 1000/180; % factor de conversión de g a mmol
 
% Comidas (perturbaciones) a lo largo de un día

Dg = 50*f;
% Ecuación
D = (Dg*Ag*(t-t1)*exp(-(t-t1)/Tmaxi))/(Vg*Tmaxg^2);

== matlab function Modelo_bergman_mod_U/Ingesta 75 g5 ==
  data: in input; D output
function D = comida(in)
% Variables de entrada en la funcion
t = in(1) %- 8*60*60; % Ajuste para iniciar a las 8 de la mañana
 
% Parámetros del modelo
Ag = 0.8; % adimensional
Tmaxi = 55*60; % s
Vg = 13.79; % L
Tmaxg = 40*60; % s
t1 = 0;
Dg = 0;
f = 1000/180; % factor de conversión de g a mmol
 
% Comidas (perturbaciones) a lo largo de un día
Dg = 50*f;
% Ecuación
D = (Dg*Ag*(t-t1)*exp(-(t-t1)/Tmaxi))/(Vg*Tmaxg^2);

== matlab function Modelo_bergman_mod_U/Ingesta 75 g6 ==
  data: in input; D output
function D = comida(in)
% Variables de entrada en la funcion
t = in(1) %- 8*60*60; % Ajuste para iniciar a las 8 de la mañana
 
% Parámetros del modelo
Ag = 0.8; % adimensional
Tmaxi = 55*60; % s
Vg = 13.79; % L
Tmaxg = 40*60; % s
t1 = 0;
Dg = 0;
f = 1000/180; % factor de conversión de g a mmol
 
% Comidas (perturbaciones) a lo largo de un día
Dg = 50*f;
 
% Ecuación
D = (Dg*Ag*(t-t1)*exp(-(t-t1)/Tmaxi))/(Vg*Tmaxg^2);

== matlab function Modelo_bergman_mod_U/Ingesta 75 g7 ==
  data: in input; D output
function D = comida(in)
% Variables de entrada en la funcion
t = in(1) %- 8*60*60; % Ajuste para iniciar a las 8 de la mañana
 
% Parámetros del modelo
Ag = 0.8; % adimensional
Tmaxi = 55*60; % s
Vg = 13.79; % L
Tmaxg = 40*60; % s
t1 = 0;
Dg = 0;
f = 1000/180; % factor de conversión de g a mmol
 
% Comidas (perturbaciones) a lo largo de un día
Dg = 50*f;
 
% Ecuación
D = (Dg*Ag*(t-t1)*exp(-(t-t1)/Tmaxi))/(Vg*Tmaxg^2);

== matlab function Modelo_bergman_mod_U/Ingesta 75 g8 ==
  data: in input; D output
function D = comida(in)
% Variables de entrada en la funcion
t = in(1) %- 8*60*60; % Ajuste para iniciar a las 8 de la mañana
 
% Parámetros del modelo
Ag = 0.8; % adimensional
Tmaxi = 55*60; % s
Vg = 13.79; % L
Tmaxg = 40*60; % s
t1 = 0;
Dg = 0;
f = 1000/180; % factor de conversión de g a mmol
 
% Comidas (perturbaciones) a lo largo de un día
Dg = 50*f;
 
% Ecuación
D = (Dg*Ag*(t-t1)*exp(-(t-t1)/Tmaxi))/(Vg*Tmaxg^2);

== matlab function Modelo_bergman_mod_U/Ingesta 75 g10 ==
  data: in input; D output
function D = comida(in)
% Variables de entrada en la funcion
t = in(1) %- 8*60*60; % Ajuste para iniciar a las 8 de la mañana
 
% Parámetros del modelo
Ag = 0.8; % adimensional
Tmaxi = 55*60; % s
Vg = 13.79; % L
Tmaxg = 40*60; % s
t1 = 0;
Dg = 0;
f = 1000/180; % factor de conversión de g a mmol
 
% Comidas (perturbaciones) a lo largo de un día
Dg = 50*f;
 
% Ecuación
D = (Dg*Ag*(t-t1)*exp(-(t-t1)/Tmaxi))/(Vg*Tmaxg^2);

== matlab function Modelo_bergman_mod_U/Ingesta 75 g9 ==
  data: in input; D output
function D = comida(in)
% Variables de entrada en la funcion
t = in(1) %- 8*60*60; % Ajuste para iniciar a las 8 de la mañana
 
% Parámetros del modelo
Ag = 0.8; % adimensional
Tmaxi = 55*60; % s
Vg = 13.79; % L
Tmaxg = 40*60; % s
t1 = 0;
Dg = 0;
f = 1000/180; % factor de conversión de g a mmol
 
% Comidas (perturbaciones) a lo largo de un día
Dg = 50*f;
 
% Ecuación
D = (Dg*Ag*(t-t1)*exp(-(t-t1)/Tmaxi))/(Vg*Tmaxg^2);

== matlab function Modelo_bergman_mod_U/Ingesta 75 g2 ==
  data: in input; D output
function D = comida(in)
% Variables de entrada en la funcion
t = in(1) %- 8*60*60; % Ajuste para iniciar a las 8 de la mañana
 
% Parámetros del modelo
Ag = 0.8; % adimensional
Tmaxi = 55*60; % s
Vg = 13.79; % L
Tmaxg = 40*60; % s
t1 = 0;
Dg = 0;
f = 1000/180; % factor de conversión de g a mmol
 
% Comidas (perturbaciones) a lo largo de un día
Dg = 50*f;
 
% Ecuación
D = (Dg*Ag*(t-t1)*exp(-(t-t1)/Tmaxi))/(Vg*Tmaxg^2);
